simulink model "NominalEncounter"  (R2018b)
settings: Solver=ode45  StartTime=0.0  StopTime=600  RelTol=1e-3  EnableMultiTasking=on
libraries: simulink x4, CalcMinDist x3, NominalTrajectory x2, BasicAircraftDynamicsBlock x2, FlattenAircraftEstimateBus x2, PerfectSurveillanceBlock x2, SLoWCBlock x1, WellClearMetricsBlock x1, StopConditionsBlock x1
settings Model: Creator=JO20596  LastModifiedBy=BI28030
settings DataIOCC: LimitDataPoints=on  MaxDataPoints=10000  SignalLoggingSaveFormat=ModelDataLogs  SaveState=on  StateSaveName=xoutNew  OutputSaveName=youtNew
settings OptimizationCC: ExpressionDepthLimit=2147483647  LifeSpan=inf
settings DebuggingCC: UnderspecifiedInitializationDetection=Classic  MergeDetectMultiDrivingBlocksExec=none  SolverPrmCheckMsg=warning  FcnCallInpInsideContextMsg=warning  StateNameClashWarn=warning  SFUnexpectedBacktrackingDiag=warning  SFNoUnconditionalDefaultTransitionDiag=warning  SFExecutionAtInitializationDiag=none
settings HardwareCC: ProdBitPerPointer=32  ProdBitPerSizeT=32  ProdBitPerPtrDiffT=32  ProdLargestAtomicFloat=None  ProdIntDivRoundTo=Undefined  ProdEndianess=Unspecified  ProdWordSize=32  ProdHWDeviceType=32-bit Generic
settings ModelReferenceCC: PropagateSignalLabelsOutOfModel=off
settings SFSimCC: SimUseLocalCustomCode=off
settings RTWCC: RTWUseLocalCustomCode=off
settings CodeAppCC: StateflowObjectComments=on
settings GRTTargetCC: TargetLangStandard=C89/C90 (ANSI)  GeneratePreprocessorConditionals=Disable all  CombineOutputUpdateFcns=off  GRTInterface=on
settings ConfigComp: CovMetricSettings=dw  CovHtmlReporting=on  CovSaveCumulativeToWorkspaceVar=on  CovSaveSingleToWorkspaceVar=on  CovExternalEMLEnable=off

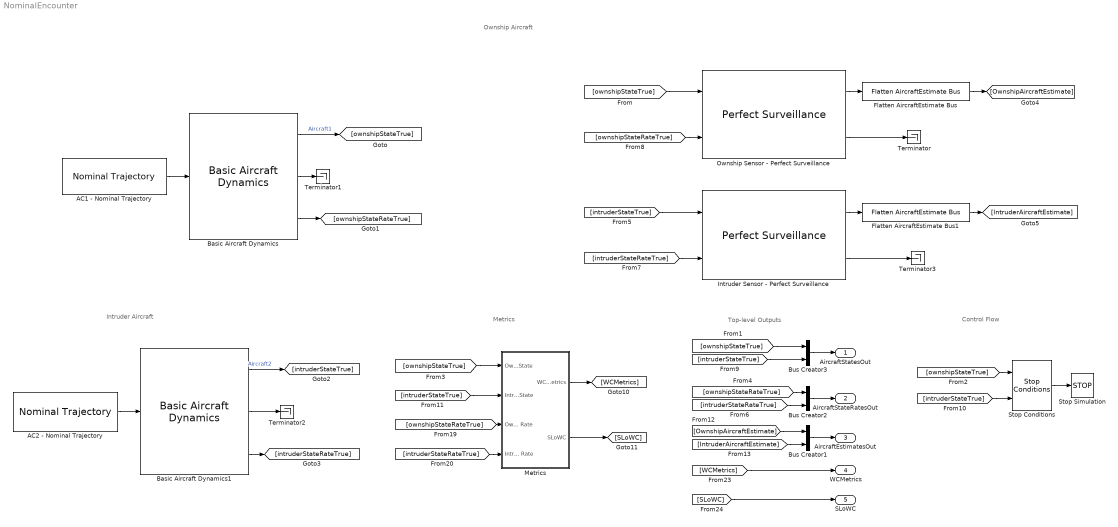
== system NominalEncounter ==
  note: Metrics
  note: Control Flow
  note: Top-level Outputs
  note: Ownship Aircraft
  note: Intruder Aircraft
  AC1 - Nominal Trajectory : NominalTrajectory/Nominal Trajectory  eventFilename=event1.mat  ts=.1
  AC2 - Nominal Trajectory : NominalTrajectory/Nominal Trajectory  eventFilename=event2.mat  ts=.1
  Basic Aircraft Dynamics : BasicAircraftDynamicsBlock/Basic Aircraft Dynamics  ts_dynamics=.1  v_ftps_0=ac1dyn_v_ftps  N_ft_0=ac1dyn_N_ft  E_ft_0=ac1dyn_E_ft  h_ft_0=ac1dyn_h_ft  psi_rad_0=ac1dyn_psi_rad  theta_rad_0=ac1dyn_theta_rad  phi_rad_0=ac1dyn_phi_rad  a_ftpss_0=ac1dyn_a_ftpss  v_ftps_max=ac1dyn_con.maxAirspeed_ftps  v_ftps_min=ac1dyn_con.minAirspeed_ftps  dv_ftpss_max=ac1dyn_con.maxAcceleration_ftpss  dv_ftpss_min=ac1dyn_con.minAcceleration_ftpss  dh_ftps_max=ac1dyn_con.maxVerticalRate_ftps  dh_ftps_min=ac1dyn_con.minVerticalRate_ftps  q_radps_max=ac1dyn_con.maxPitchRate_radps  phi_rad_max=ac1dyn_con.maxBankAngle_rad  dphi_radps_max=ac1dyn_con.maxRollRate_radps  r_radps_max=ac1dyn_con.maxYawRate_radps  pNUM=ac1dyn_con.dynamicsNumeratorRollRate  pDEN=ac1dyn_con.dynamicsDenominatorRollRate  hNUM=ac1dyn_con.dynamicsNumeratorVerticalRate  hDEN=ac1dyn_con.dynamicsDenominatorVerticalRate  rNUM=ac1dyn_con.dynamicsNumeratorYawRate  rDEN=ac1dyn_con.dynamicsDenominatorYawRate  lat0_rad=ac1dyn_lat0_rad  lon0_rad=ac1dyn_lon0_rad  alt_ft=ac1dyn_alt0_ft
  Basic Aircraft Dynamics1 : BasicAircraftDynamicsBlock/Basic Aircraft Dynamics  ts_dynamics=.1  v_ftps_0=ac2dyn_v_ftps  N_ft_0=ac2dyn_N_ft  E_ft_0=ac2dyn_E_ft  h_ft_0=ac2dyn_h_ft  psi_rad_0=ac2dyn_psi_rad  theta_rad_0=ac2dyn_theta_rad  phi_rad_0=ac2dyn_phi_rad  a_ftpss_0=ac2dyn_a_ftpss  v_ftps_max=ac2dyn_con.maxAirspeed_ftps  v_ftps_min=ac2dyn_con.minAirspeed_ftps  dv_ftpss_max=ac2dyn_con.maxAcceleration_ftpss  dv_ftpss_min=ac2dyn_con.minAcceleration_ftpss  dh_ftps_max=ac2dyn_con.maxVerticalRate_ftps  dh_ftps_min=ac2dyn_con.minVerticalRate_ftps  q_radps_max=ac2dyn_con.maxPitchRate_radps  phi_rad_max=ac2dyn_con.maxBankAngle_rad  dphi_radps_max=ac2dyn_con.maxRollRate_radps  r_radps_max=ac2dyn_con.maxYawRate_radps  pNUM=ac2dyn_con.dynamicsNumeratorRollRate  pDEN=ac2dyn_con.dynamicsDenominatorRollRate  hNUM=ac2dyn_con.dynamicsNumeratorVerticalRate  hDEN=ac2dyn_con.dynamicsDenominatorVerticalRate  rNUM=ac2dyn_con.dynamicsNumeratorYawRate  rDEN=ac2dyn_con.dynamicsDenominatorYawRate  lat0_rad=ac2dyn_lat0_rad  lon0_rad=ac2dyn_lon0_rad  alt_ft=ac2dyn_alt0_ft
  Bus Creator1 : BusCreator  Inputs=2
  Bus Creator2 : BusCreator  Inputs=2
  Bus Creator3 : BusCreator  Inputs=2
  Flatten AircraftEstimate Bus : FlattenAircraftEstimateBus/Flatten AircraftEstimate Bus  SystemSampleTime=-1
  Flatten AircraftEstimate Bus1 : FlattenAircraftEstimateBus/Flatten AircraftEstimate Bus  SystemSampleTime=-1
  Intruder Sensor - Perfect Surveillance : PerfectSurveillanceBlock/Perfect Surveillance  Description=|  dt=ac1IntPerfSurv_surveillanceSampletime_s
      | Documentation for Perfect Observation Block                                                                                                                                                                                                                                                                                                                                                                                                          
      |                                                                                                                                                                                                                                                                                                                                                                                                                                                      
      | Description:  The perfect observation block, also known as a perfect                                                                                                                                                                                                                                                                                                                                                                                 
      | surveillance block, receives an Aircraft State, nominally from a Basic                                                                                                                                                                                                                                                                                                                                                                               
      | Aircraft Dynamics block, and outputs an Aircraft Estimate.  The Aircraft                                                                                                                                                                                                                                                                                                                                                                             
      | State that is received as input consists of Latitude, Longitude, and                                                                                                                                                                                                                                                                                                                                                                                 
      | Altitude state information as well as the aircraft position in local                                                                                                                                                                                                                                                                                                                                                                                 
      | coordinates in units of feet for north, east, and height.  The Aircraft                                                                                                                                                                                                                                                                                                                                                                              
      | Estimate outputs consist of estimates for the aircraft Latitude, Longitude, and Altitude, the east, north up position, and sensor covariance.  For perfect surveillance, the covariance estimates are all set to zero as default.  In addition, "time of validity" and a Boolean flag for the sensor report, "is Valid", are outputted as part of the Aircraft Estimate.                                                                             
      |                                                                                                                                                                                                                                                                                                                                                                                                                                                      
      | The initial perfect surveillance block developed receives the aircraft state information from the "AC2 - Basic Aircraft Dynamics" block within the "nominalEncounter" study.  Since the expected output from the AC1 and AC2 aircraft states have slightly different output parameters than what is provided from the perfect surveillance block (i.e., covariance estimates, isValid, and time of validity), the perfect surveillance block         
      | AircraftEstimate output has been left disconnected.                                                                                                                                                                                                                                                                                                                                                                                                  
      |                                                                                                                                                                                                                                                                                                                                                                                                                                                      
      | The initial unit test performed for this perfect observation block was to                                                                                                                                                                                                                                                                                                                                                                            
      | run the nominalEncounter study and to ensure that the simulation completes and no exceptions are encountered.  This unit test was successful (other than receiving a warning that the output of the perfect surveillance block is not connected, which was expected).  A more comprehensive future unit test would be to evaluate the position inputs and compare them with the position outputs to ensure that they are consistent with one another.
  Metrics : Subsystem
  Ownship Sensor - Perfect Surveillance : PerfectSurveillanceBlock/Perfect Surveillance  Description=|  dt=ac1OwnPerfSurv_surveillanceSampletime_s
      | Documentation for Perfect Observation Block                                                                                                                                                                                                                                                                                                                                                                                                          
      |                                                                                                                                                                                                                                                                                                                                                                                                                                                      
      | Description:  The perfect observation block, also known as a perfect                                                                                                                                                                                                                                                                                                                                                                                 
      | surveillance block, receives an Aircraft State, nominally from a Basic                                                                                                                                                                                                                                                                                                                                                                               
      | Aircraft Dynamics block, and outputs an Aircraft Estimate.  The Aircraft                                                                                                                                                                                                                                                                                                                                                                             
      | State that is received as input consists of Latitude, Longitude, and                                                                                                                                                                                                                                                                                                                                                                                 
      | Altitude state information as well as the aircraft position in local                                                                                                                                                                                                                                                                                                                                                                                 
      | coordinates in units of feet for north, east, and height.  The Aircraft                                                                                                                                                                                                                                                                                                                                                                              
      | Estimate outputs consist of estimates for the aircraft Latitude, Longitude, and Altitude, the east, north up position, and sensor covariance.  For perfect surveillance, the covariance estimates are all set to zero as default.  In addition, "time of validity" and a Boolean flag for the sensor report, "is Valid", are outputted as part of the Aircraft Estimate.                                                                             
      |                                                                                                                                                                                                                                                                                                                                                                                                                                                      
      | The initial perfect surveillance block developed receives the aircraft state information from the "AC2 - Basic Aircraft Dynamics" block within the "nominalEncounter" study.  Since the expected output from the AC1 and AC2 aircraft states have slightly different output parameters than what is provided from the perfect surveillance block (i.e., covariance estimates, isValid, and time of validity), the perfect surveillance block         
      | AircraftEstimate output has been left disconnected.                                                                                                                                                                                                                                                                                                                                                                                                  
      |                                                                                                                                                                                                                                                                                                                                                                                                                                                      
      | The initial unit test performed for this perfect observation block was to                                                                                                                                                                                                                                                                                                                                                                            
      | run the nominalEncounter study and to ensure that the simulation completes and no exceptions are encountered.  This unit test was successful (other than receiving a warning that the output of the perfect surveillance block is not connected, which was expected).  A more comprehensive future unit test would be to evaluate the position inputs and compare them with the position outputs to ensure that they are consistent with one another.
  Stop Conditions : StopConditionsBlock/Stop Conditions  range_limit_ft=stop_range_ft  altitude_limit_ft=stop_altitude_ft
  Stop Simulation : Stop
  Terminator{,1..3} (4 alike) : Terminator
  AircraftStatesOut : Outport
  AircraftStateRatesOut : Outport  Port=2
  AircraftEstimatesOut : Outport  Port=3
  WCMetrics : Outport  Port=4
  SLoWC : Outport  Port=5
  wires:
  Bus Creator2/1 -> AircraftStateRatesOut/1
  Stop Conditions/1 -> Stop Simulation/1
  [ownshipStateTrue] -> Stop Conditions/1
  [ownshipStateRateTrue] -> Bus Creator2/1
  [intruderStateRateTrue] -> Bus Creator2/2
  [intruderStateTrue] -> Stop Conditions/2
  [ownshipStateTrue] -> Metrics/1(Ownship State)
  [intruderStateTrue] -> Metrics/2(Intruder State)
  [ownshipStateRateTrue] -> Metrics/3(Ownship State Rate)
  [intruderStateRateTrue] -> Metrics/4(Intruder State Rate)
  Metrics/1(WCMetrics) -> [WCMetrics]
  Metrics/2(SLoWC) -> [SLoWC]
  [WCMetrics] -> WCMetrics/1
  [SLoWC] -> SLoWC/1
  Basic Aircraft Dynamics1/3 -> [intruderStateRateTrue]
  Basic Aircraft Dynamics/2 -> Terminator1/1
  AC1 - Nominal Trajectory/1 -> Basic Aircraft Dynamics/1
  Basic Aircraft Dynamics1/1 -> [intruderStateTrue]  "Aircraft2"
  Basic Aircraft Dynamics1/2 -> Terminator2/1
  AC2 - Nominal Trajectory/1 -> Basic Aircraft Dynamics1/1
  Basic Aircraft Dynamics/1 -> [ownshipStateTrue]  "Aircraft1"
  [ownshipStateTrue] -> Ownship Sensor - Perfect Surveillance/1
  Basic Aircraft Dynamics/3 -> [ownshipStateRateTrue]
  [intruderStateTrue] -> Intruder Sensor - Perfect Surveillance/1
  [intruderStateRateTrue] -> Intruder Sensor - Perfect Surveillance/2
  [ownshipStateRateTrue] -> Ownship Sensor - Perfect Surveillance/2
  [OwnshipAircraftEstimate] -> Bus Creator1/1
  [IntruderAircraftEstimate] -> Bus Creator1/2
  Ownship Sensor - Perfect Surveillance/1 -> Flatten AircraftEstimate Bus/1
  Intruder Sensor - Perfect Surveillance/1 -> Flatten AircraftEstimate Bus1/1
  Bus Creator1/1 -> AircraftEstimatesOut/1
  Flatten AircraftEstimate Bus1/1 -> [IntruderAircraftEstimate]
  Flatten AircraftEstimate Bus/1 -> [OwnshipAircraftEstimate]
  [ownshipStateTrue] -> Bus Creator3/1
  [intruderStateTrue] -> Bus Creator3/2
  Bus Creator3/1 -> AircraftStatesOut/1
  Ownship Sensor - Perfect Surveillance/2 -> Terminator/1
  Intruder Sensor - Perfect Surveillance/2 -> Terminator3/1

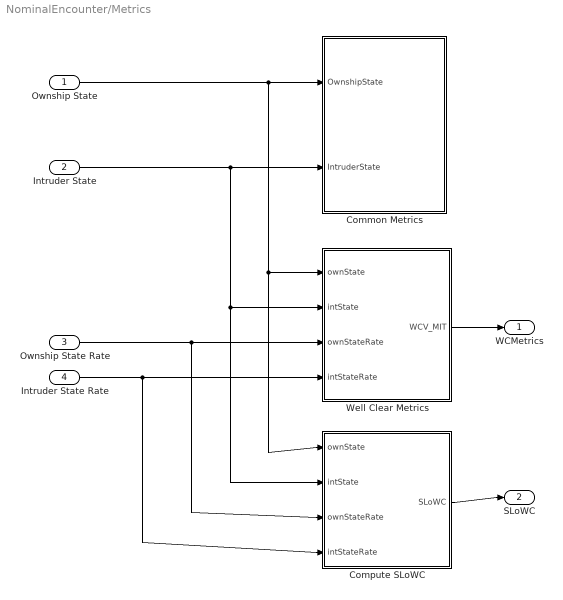
== system NominalEncounter/Metrics ==
  Ownship State : Inport
  Intruder State : Inport  Port=2
  Ownship State Rate : Inport  Port=3
  Intruder State Rate : Inport  Port=4
  Common Metrics : Subsystem  AncestorBlock=CommonMetricsBlock/Common Metrics  mask(CommonMetrics){}
      mask help:
      | Calculates metrics common to all aircraft encounters, those having to do with the separation
      | between aircraft. Metrics pertaining to the operation of advisory systems (e.g. alert rate) are not
      | included in this block.
      |
      | The calculated metrics are saved to a workspace.
      mask Help:
      | Calculates metrics common to all aircraft encounters, those having to do with the separation
      | between aircraft. Metrics pertaining to the operation of advisory systems (e.g. alert rate) are not
      | included in this block.
      | 
      | The calculated metrics are saved to a workspace.
      | 
      | INPUTS
      | ==========
      | Aircraft1 - A CASSATT v6 AircraftState bus from first aircraft
      | Aircraft2 - A CASSATT v6 AircraftState bus from second aircraft
      | 
      | OUTPUTS (Saved to Workspace)
      | ==========
      | NMAC - Near Mid Air Collision.  True if the separation between the two
      |     aircraft has ever been simultaneously less than 100 feet vertically and
      |     500 feet horizontally.
      | hmd_ft - Horizontal Miss Distance in feet.  The minimum horizontal
      |     separation that has occurred between the two aircraft.
      | vmd_ft - Vertical Miss Distance in feet.  The vertical separation of the
      |     two aircaft at the Time of Closest Approach.
      | tca - Time of Closest Approach in seconds.  Prior to horizontal separation
      |     of less than 500 feet, the Time of Closest Approach is the time when
      |     the minimum horizontal separation was achieved.  Once horizontal
      |     separation has been less than 500 feet, the Time of Closest Approach is
      |     when minimum vertical separation occurs while horizontal separation is
      |     less than 500 feet.
  Compute SLoWC : Subsystem  mask{DMOD=4000, tauMod=35, altDiff=450}
      mask prompts: altDiff "Altitude Difference Threshold:"
  Well Clear Metrics : Subsystem
  WCMetrics : Outport
  SLoWC : Outport  Port=2
  wires:
  Ownship State/1 -> Common Metrics/1(OwnshipState), Well Clear Metrics/1(ownState), Compute SLoWC/1(ownState)
  Intruder State/1 -> Common Metrics/2(IntruderState), Well Clear Metrics/2(intState), Compute SLoWC/2(intState)
  Ownship State Rate/1 -> Well Clear Metrics/3(ownStateRate), Compute SLoWC/3(ownStateRate)
  Intruder State Rate/1 -> Well Clear Metrics/4(intStateRate), Compute SLoWC/4(intStateRate)
  Well Clear Metrics/1(WCV_MIT) -> WCMetrics/1
  Compute SLoWC/1(SLoWC) -> SLoWC/1

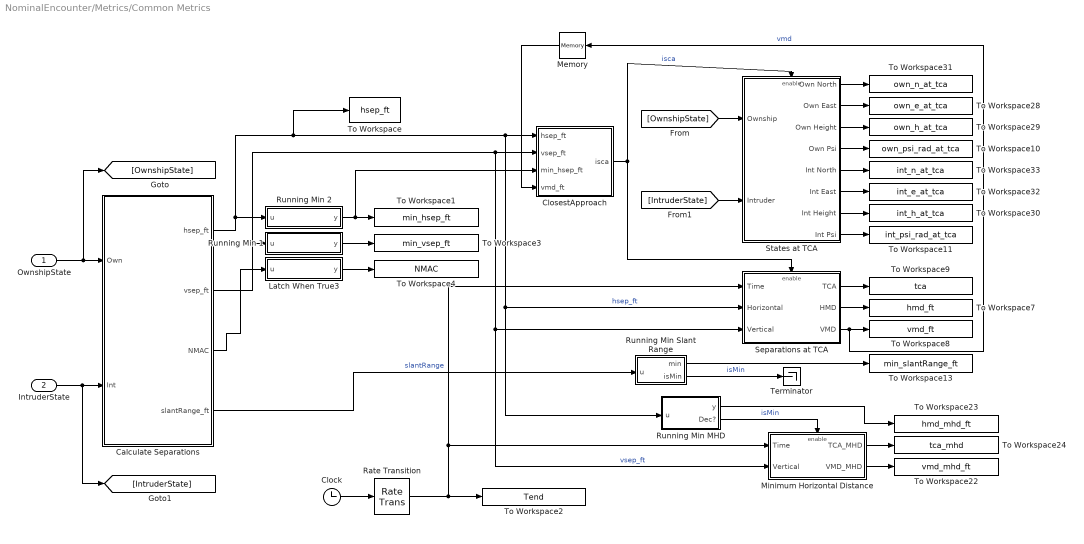
== system NominalEncounter/Metrics/Common Metrics ==
  OwnshipState : Inport  OutDataTypeStr=Bus: AircraftState  PortDimensions=1
  IntruderState : Inport  Port=2  OutDataTypeStr=Bus: AircraftState  PortDimensions=1
  Calculate Separations : Subsystem
  Clock : Clock
  ClosestApproach : Subsystem
  Latch When True3 : Subsystem
      mask Display: disp('Latch when true')
  Memory : Memory
  Minimum Horizontal Distance : Subsystem  TreatAsAtomicUnit=on
  Rate Transition : RateTransition
  Running Min 1 : Subsystem
      mask Display: disp('Running min')
  Running Min 2 : Subsystem
      mask Display: disp('Running min')
  Running Min MHD : Subsystem
  Running Min Slant Range : Subsystem
  Separations at TCA : Subsystem  TreatAsAtomicUnit=on
  States at TCA : Subsystem  TreatAsAtomicUnit=on
  Terminator : Terminator
  To Workspace : ToWorkspace  VariableName=hsep_ft  SaveFormat=Timeseries  SampleTime=-1
  To Workspace1 : ToWorkspace  VariableName=min_hsep_ft  SampleTime=-1
      settings: MaxDataPoints=1
  To Workspace10 : ToWorkspace  VariableName=own_psi_rad_at_tca  SampleTime=-1
      settings: MaxDataPoints=1
  To Workspace11 : ToWorkspace  VariableName=int_psi_rad_at_tca  SampleTime=-1
      settings: MaxDataPoints=1
  To Workspace13 : ToWorkspace  VariableName=min_slantRange_ft  SampleTime=-1
      settings: MaxDataPoints=1
  To Workspace2 : ToWorkspace  VariableName=Tend  SampleTime=-1
      settings: MaxDataPoints=1
  To Workspace22 : ToWorkspace  VariableName=vmd_mhd_ft  SampleTime=-1
      settings: MaxDataPoints=1
  To Workspace23 : ToWorkspace  VariableName=hmd_mhd_ft  SampleTime=-1
      settings: MaxDataPoints=1
  To Workspace24 : ToWorkspace  VariableName=tca_mhd  SampleTime=-1
      settings: MaxDataPoints=1
  To Workspace28 : ToWorkspace  VariableName=own_e_at_tca  SampleTime=-1
      settings: MaxDataPoints=1
  To Workspace29 : ToWorkspace  VariableName=own_h_at_tca  SampleTime=-1
      settings: MaxDataPoints=1
  To Workspace3 : ToWorkspace  VariableName=min_vsep_ft  SampleTime=-1
      settings: MaxDataPoints=1
  To Workspace30 : ToWorkspace  VariableName=int_h_at_tca  SampleTime=-1
      settings: MaxDataPoints=1
  To Workspace31 : ToWorkspace  VariableName=own_n_at_tca  SampleTime=-1
      settings: MaxDataPoints=1
  To Workspace32 : ToWorkspace  VariableName=int_e_at_tca  SampleTime=-1
      settings: MaxDataPoints=1
  To Workspace33 : ToWorkspace  VariableName=int_n_at_tca  SampleTime=-1
      settings: MaxDataPoints=1
  To Workspace4 : ToWorkspace  VariableName=NMAC  SampleTime=-1
      settings: MaxDataPoints=1
  To Workspace7 : ToWorkspace  VariableName=hmd_ft  SampleTime=-1
      settings: MaxDataPoints=1
  To Workspace8 : ToWorkspace  VariableName=vmd_ft  SampleTime=-1
      settings: MaxDataPoints=1
  To Workspace9 : ToWorkspace  VariableName=tca  SampleTime=-1
      settings: MaxDataPoints=1
  wires:
  Calculate Separations/2(vsep_ft) -> ClosestApproach/2(vsep_ft), Separations at TCA/3(Vertical), Minimum Horizontal Distance/2(Vertical), Running Min 1/1(u)  "vsep_ft"
  Rate Transition/1 -> To Workspace2/1, Separations at TCA/1(Time), Minimum Horizontal Distance/1(Time)
  Minimum Horizontal Distance/1(TCA_MHD) -> To Workspace24/1
  Minimum Horizontal Distance/2(VMD_MHD) -> To Workspace22/1
  Running Min MHD/1(y) -> To Workspace23/1
  Running Min MHD/2(Dec?) -> Minimum Horizontal Distance/Enable  "isMin"
  Running Min Slant Range/2(isMin) -> Terminator/1  "isMin"
  Running Min 2/1(y) -> To Workspace1/1, ClosestApproach/3(min_hsep_ft)
  Separations at TCA/3(VMD) -> To Workspace8/1, Memory/1  "vmd"
  Clock/1 -> Rate Transition/1
  Separations at TCA/1(TCA) -> To Workspace9/1
  Latch When True3/1(y) -> To Workspace4/1
  IntruderState/1 -> Calculate Separations/2(Int), [IntruderState]
  Calculate Separations/3(NMAC) -> Latch When True3/1(u)
  Separations at TCA/2(HMD) -> To Workspace7/1
  Running Min 1/1(y) -> To Workspace3/1
  Calculate Separations/4(slantRange_ft) -> Running Min Slant Range/1(u)  "slantRange"
  Running Min Slant Range/1(min) -> To Workspace13/1
  Calculate Separations/1(hsep_ft) -> Running Min 2/1(u), To Workspace/1, ClosestApproach/1(hsep_ft), Separations at TCA/2(Horizontal), Running Min MHD/1(u)  "hsep_ft"
  ClosestApproach/1(isca) -> Separations at TCA/Enable, States at TCA/Enable  "isca"
  States at TCA/1(Own North) -> To Workspace31/1
  States at TCA/2(Own East) -> To Workspace28/1
  States at TCA/3(Own Height) -> To Workspace29/1
  States at TCA/5(Int North) -> To Workspace33/1
  States at TCA/6(Int East) -> To Workspace32/1
  States at TCA/7(Int Height) -> To Workspace30/1
  [OwnshipState] -> States at TCA/1(Ownship)
  [IntruderState] -> States at TCA/2(Intruder)
  OwnshipState/1 -> Calculate Separations/1(Own), [OwnshipState]
  Memory/1 -> ClosestApproach/4(vmd_ft)
  States at TCA/4(Own Psi) -> To Workspace10/1
  States at TCA/8(Int Psi) -> To Workspace11/1

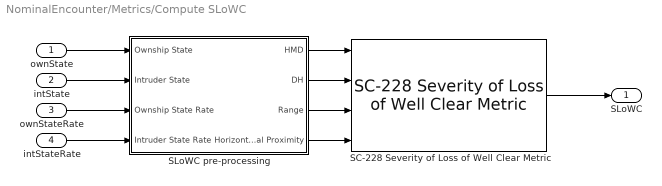
== system NominalEncounter/Metrics/Compute SLoWC ==
  ownState : Inport
  intState : Inport  Port=2
  ownStateRate : Inport  Port=3
  intStateRate : Inport  Port=4
  SC-228 Severity of Loss of Well Clear Metric : SLoWCBlock/SC-228 Severity of Loss of Well Clear Metric  DMOD=DMOD  altDiffThreshold=altDiff
  SLoWC pre-processing : Subsystem
  SLoWC : Outport
  wires:
  SLoWC pre-processing/2(DH) -> SC-228 Severity of Loss of Well Clear Metric/2
  SC-228 Severity of Loss of Well Clear Metric/1 -> SLoWC/1
  SLoWC pre-processing/1(HMD) -> SC-228 Severity of Loss of Well Clear Metric/1
  ownState/1 -> SLoWC pre-processing/1(Ownship State)
  SLoWC pre-processing/4(Horizontal Proximity) -> SC-228 Severity of Loss of Well Clear Metric/4
  SLoWC pre-processing/3(Range) -> SC-228 Severity of Loss of Well Clear Metric/3
  intState/1 -> SLoWC pre-processing/2(Intruder State)
  intStateRate/1 -> SLoWC pre-processing/4(Intruder State Rate)
  ownStateRate/1 -> SLoWC pre-processing/3(Ownship State Rate)

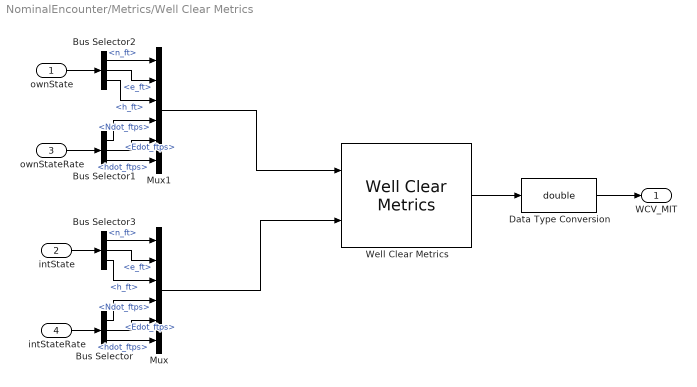
== system NominalEncounter/Metrics/Well Clear Metrics ==
  ownState : Inport  OutDataTypeStr=Bus: AircraftState
  intState : Inport  Port=2  OutDataTypeStr=Bus: AircraftState
  ownStateRate : Inport  Port=3  OutDataTypeStr=Bus: AircraftStateRate
  intStateRate : Inport  Port=4  OutDataTypeStr=Bus: AircraftStateRate
  Bus Selector : BusSelector  OutputSignals=Ndot_ftps,Edot_ftps,hdot_ftps
  Bus Selector1 : BusSelector  OutputSignals=Ndot_ftps,Edot_ftps,hdot_ftps
  Bus Selector2 : BusSelector  OutputSignals=n_ft,e_ft,h_ft
  Bus Selector3 : BusSelector  OutputSignals=n_ft,e_ft,h_ft
  Data Type Conversion : DataTypeConversion  OutDataTypeStr=double
  Mux : Mux  Inputs=6
  Mux1 : Mux  Inputs=6
  Well Clear Metrics : WellClearMetricsBlock/Well Clear Metrics  tauThreshold=wcm_modTau  hmdThreshold=wcm_HMD  tauVThreshold=wcm_TOCA  altThreshold=wcm_altThresh  rngThreshold=wcm_rangeThresh
  WCV_MIT : Outport
  wires:
  Well Clear Metrics/1 -> Data Type Conversion/1
  intStateRate/1 -> Bus Selector/1
  ownStateRate/1 -> Bus Selector1/1
  ownState/1 -> Bus Selector2/1
  intState/1 -> Bus Selector3/1
  Bus Selector3/1 -> Mux/1  "<n_ft>"
  Bus Selector3/2 -> Mux/2  "<e_ft>"
  Bus Selector3/3 -> Mux/3  "<h_ft>"
  Bus Selector/1 -> Mux/4  "<Ndot_ftps>"
  Bus Selector/2 -> Mux/5  "<Edot_ftps>"
  Bus Selector/3 -> Mux/6  "<hdot_ftps>"
  Bus Selector2/1 -> Mux1/1  "<n_ft>"
  Bus Selector2/2 -> Mux1/2  "<e_ft>"
  Bus Selector2/3 -> Mux1/3  "<h_ft>"
  Bus Selector1/3 -> Mux1/6  "<hdot_ftps>"
  Bus Selector1/1 -> Mux1/4  "<Ndot_ftps>"
  Bus Selector1/2 -> Mux1/5  "<Edot_ftps>"
  Mux1/1 -> Well Clear Metrics/1
  Mux/1 -> Well Clear Metrics/2
  Data Type Conversion/1 -> WCV_MIT/1

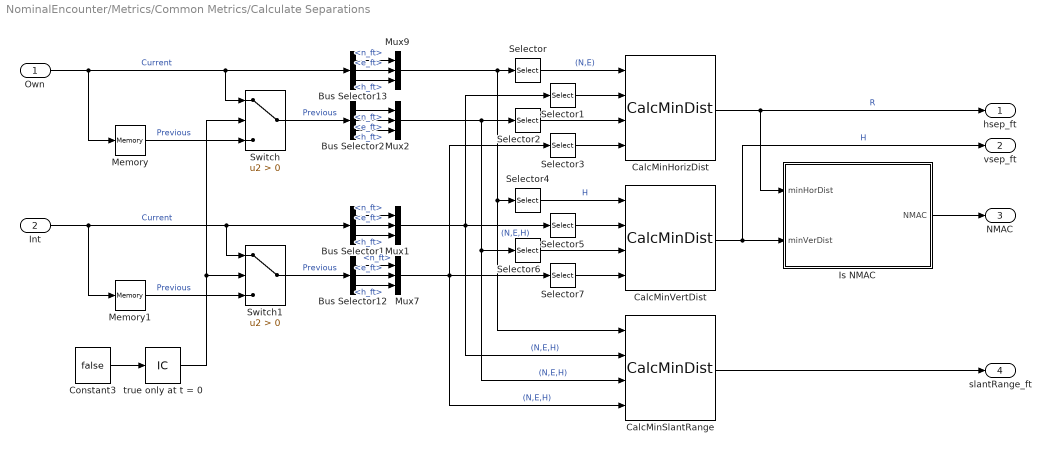
== system NominalEncounter/Metrics/Common Metrics/Calculate Separations ==
  Own : Inport
  Int : Inport  Port=2
  Bus Selector{1..2,12..13} (4 alike) : BusSelector  OutputSignals=n_ft,e_ft,h_ft
  CalcMinHorizDist : CalcMinDist/CalcMinDist
      settings: SourceProductName=CASSATTv6: Metrics Library
  CalcMinSlantRange : CalcMinDist/CalcMinDist
      settings: SourceProductName=CASSATTv6: Metrics Library
  CalcMinVertDist : CalcMinDist/CalcMinDist
      settings: SourceProductName=CASSATTv6: Metrics Library
  Constant3 : Constant  Value=false  SampleTime=Inf
  Is NMAC : Subsystem
  Memory : Memory
  Memory1 : Memory
  Mux{1..2,7,9} (4 alike) : Mux  Inputs=3
  Selector{,1..3} (4 alike) : Selector  InputPortWidth=3  IndexOptions=Index vector (dialog)  Indices=[1 2]  OutputSizes=1
  Selector{4..7} (4 alike) : Selector  InputPortWidth=3  IndexOptions=Index vector (dialog)  Indices=3  OutputSizes=1
  Switch : Switch  Criteria=u2 > Threshold
  Switch1 : Switch  Criteria=u2 > Threshold
  true only at t = 0 : InitialCondition  Value=true
  hsep_ft : Outport
  vsep_ft : Outport  Port=2
  NMAC : Outport  Port=3
  slantRange_ft : Outport  Port=4
  wires:
  CalcMinHorizDist/1 -> Is NMAC/1(minHorDist), hsep_ft/1  "R"
  true only at t = 0/1 -> Switch/2, Switch1/2
  Constant3/1 -> true only at t = 0/1
  Memory1/1 -> Switch1/3  "Previous"
  Memory/1 -> Switch/3  "Previous"
  Mux9/1 -> Selector/1, Selector4/1, CalcMinSlantRange/1  "(N,E,H)"
  Bus Selector12/2 -> Mux7/2  "<e_ft>"
  Bus Selector12/1 -> Mux7/1  "<n_ft>"
  Bus Selector12/3 -> Mux7/3  "<h_ft>"
  Mux7/1 -> Selector3/1, Selector7/1, CalcMinSlantRange/4  "(N,E,H)"
  CalcMinSlantRange/1 -> slantRange_ft/1
  Int/1 -> Bus Selector1/1, Switch1/1, Memory1/1  "Current"
  Own/1 -> Memory/1, Bus Selector13/1, Switch/1  "Current"
  Switch1/1 -> Bus Selector12/1  "Previous"
  CalcMinVertDist/1 -> vsep_ft/1, Is NMAC/2(minVerDist)  "H"
  Bus Selector13/1 -> Mux9/1  "<n_ft>"
  Bus Selector13/2 -> Mux9/2  "<e_ft>"
  Bus Selector13/3 -> Mux9/3  "<h_ft>"
  Bus Selector1/1 -> Mux1/1  "<n_ft>"
  Bus Selector1/2 -> Mux1/2  "<e_ft>"
  Bus Selector1/3 -> Mux1/3  "<h_ft>"
  Switch/1 -> Bus Selector2/1  "Previous"
  Bus Selector2/1 -> Mux2/1  "<n_ft>"
  Bus Selector2/2 -> Mux2/2  "<e_ft>"
  Bus Selector2/3 -> Mux2/3  "<h_ft>"
  Mux1/1 -> Selector1/1, Selector5/1, CalcMinSlantRange/2  "(N,E,H)"
  Mux2/1 -> Selector6/1, CalcMinSlantRange/3, Selector2/1  "(N,E,H)"
  Selector/1 -> CalcMinHorizDist/1  "(N,E)"
  Selector1/1 -> CalcMinHorizDist/2
  Selector2/1 -> CalcMinHorizDist/3
  Selector3/1 -> CalcMinHorizDist/4
  Selector4/1 -> CalcMinVertDist/1  "H"
  Selector5/1 -> CalcMinVertDist/2
  Selector6/1 -> CalcMinVertDist/3
  Selector7/1 -> CalcMinVertDist/4
  Is NMAC/1(NMAC) -> NMAC/1

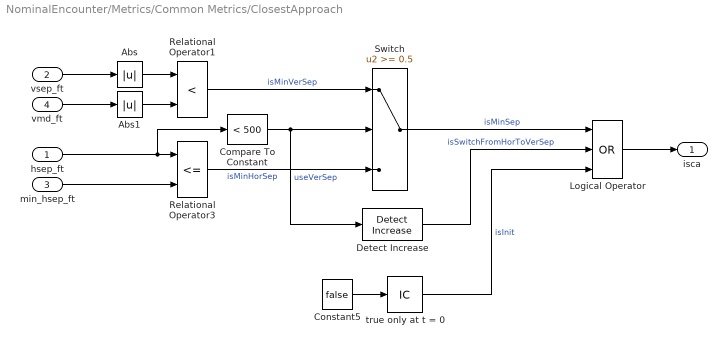
== system NominalEncounter/Metrics/Common Metrics/ClosestApproach ==
  hsep_ft : Inport
  vsep_ft : Inport  Port=2
  min_hsep_ft : Inport  Port=3
  vmd_ft : Inport  Port=4
  Abs : Abs
  Abs1 : Abs
  Compare To Constant : simulink/Logic and Bit Operations/Compare To Constant  relop=<  const=500  OutDataTypeStr=boolean
  Constant5 : Constant  Value=false  SampleTime=Inf
  Detect Increase : simulink/Logic and Bit Operations/Detect Increase  vinit=0.0  OutDataTypeStr=boolean
  Logical Operator : Logic  Operator=OR  Inputs=3  AllPortsSameDT=off  OutDataTypeStr=boolean
  Relational Operator1 : RelationalOperator  Operator=<  OutDataTypeStr=boolean  RndMeth=Nearest
  Relational Operator3 : RelationalOperator  Operator=<=  OutDataTypeStr=boolean  RndMeth=Nearest
  Switch : Switch  Threshold=0.5
  true only at t = 0 : InitialCondition  Value=true
  isca : Outport
  wires:
  Detect Increase/1 -> Logical Operator/2  "isSwitchFromHorToVerSep"
  Logical Operator/1 -> isca/1
  hsep_ft/1 -> Compare To Constant/1, Relational Operator3/1
  Compare To Constant/1 -> Switch/2, Detect Increase/1  "useVerSep"
  Switch/1 -> Logical Operator/1  "isMinSep"
  vsep_ft/1 -> Abs/1
  vmd_ft/1 -> Abs1/1
  Abs1/1 -> Relational Operator1/2
  Abs/1 -> Relational Operator1/1
  Relational Operator1/1 -> Switch/1  "isMinVerSep"
  min_hsep_ft/1 -> Relational Operator3/2
  Relational Operator3/1 -> Switch/3  "isMinHorSep"
  Constant5/1 -> true only at t = 0/1
  true only at t = 0/1 -> Logical Operator/3  "isInit"

== system NominalEncounter/Metrics/Common Metrics/Latch When True3 ==
  u : Inport  PortDimensions=1
  Logical Operator : Logic  Operator=OR  AllPortsSameDT=off  OutDataTypeStr=boolean
  Unit Delay : UnitDelay  SampleTime=-1
  y : Outport
  wires:
  Unit Delay/1 -> Logical Operator/2
  Logical Operator/1 -> Unit Delay/1, y/1
  u/1 -> Logical Operator/1

== system NominalEncounter/Metrics/Common Metrics/Minimum Horizontal Distance ==
  note: This subsytems passes the input signal through whenever the enable signal is true. The output is held when the enable signal is false.
  Time : Inport
  Vertical : Inport  Port=2
  isca : EnablePort
  TCA_MHD : Outport
  VMD_MHD : Outport  Port=2
  wires:
  Vertical/1 -> VMD_MHD/1
  Time/1 -> TCA_MHD/1

== system NominalEncounter/Metrics/Common Metrics/Running Min 1 ==
  u : Inport  PortDimensions=1
  MinMax : MinMax  Inputs=2
  Unit Delay : UnitDelay  InitialCondition=NaN  SampleTime=-1
  y : Outport
  wires:
  u/1 -> MinMax/1
  MinMax/1 -> y/1, Unit Delay/1
  Unit Delay/1 -> MinMax/2

== system NominalEncounter/Metrics/Common Metrics/Running Min 2 ==
  u : Inport  PortDimensions=1
  MinMax : MinMax  Inputs=2
  Unit Delay : UnitDelay  InitialCondition=NaN  SampleTime=-1
  y : Outport
  wires:
  Unit Delay/1 -> MinMax/2
  MinMax/1 -> Unit Delay/1, y/1
  u/1 -> MinMax/1

== system NominalEncounter/Metrics/Common Metrics/Running Min MHD ==
  u : Inport
  Memory : Memory  InitialCondition=42000000
  Relational Operator : RelationalOperator  Operator=<=  OutDataTypeStr=boolean  RndMeth=Nearest
  Switch : Switch  Criteria=u2 ~= 0
  y : Outport
  Dec? : Outport  Port=2
  wires:
  Relational Operator/1 -> Switch/2, Dec?/1
  u/1 -> Relational Operator/1, Switch/1
  Memory/1 -> Relational Operator/2, Switch/3
  Switch/1 -> Memory/1, y/1

== system NominalEncounter/Metrics/Common Metrics/Running Min Slant Range ==
  u : Inport
  MinMax : MinMax  Inputs=2
  Relational Operator : RelationalOperator  Operator=<=  OutDataTypeStr=boolean  RndMeth=Nearest
  Unit Delay : UnitDelay  InitialCondition=inf  SampleTime=-1
  min : Outport
  isMin : Outport  Port=2
  wires:
  Relational Operator/1 -> isMin/1
  Unit Delay/1 -> MinMax/2, Relational Operator/2  "old value"
  MinMax/1 -> Unit Delay/1, min/1
  u/1 -> Relational Operator/1, MinMax/1  "new value"

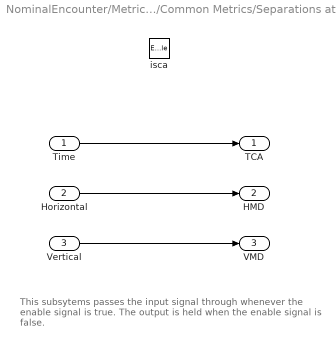
== system NominalEncounter/Metrics/Common Metrics/Separations at TCA ==
  note: This subsytems passes the input signal through whenever the enable signal is true. The output is held when the enable signal is false.
  Time : Inport
  Horizontal : Inport  Port=2
  Vertical : Inport  Port=3
  isca : EnablePort
  TCA : Outport
  HMD : Outport  Port=2
  VMD : Outport  Port=3
  wires:
  Time/1 -> TCA/1
  Horizontal/1 -> HMD/1
  Vertical/1 -> VMD/1

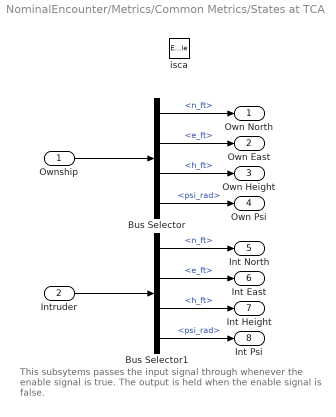
== system NominalEncounter/Metrics/Common Metrics/States at TCA ==
  note: This subsytems passes the input signal through whenever the enable signal is true. The output is held when the enable signal is false.
  Ownship : Inport
  Intruder : Inport  Port=2
  isca : EnablePort
  Bus Selector : BusSelector  OutputSignals=n_ft,e_ft,h_ft,psi_rad
  Bus Selector1 : BusSelector  OutputSignals=n_ft,e_ft,h_ft,psi_rad
  Own North : Outport
  Own East : Outport  Port=2
  Own Height : Outport  Port=3
  Own Psi : Outport  Port=4
  Int North : Outport  Port=5
  Int East : Outport  Port=6
  Int Height : Outport  Port=7
  Int Psi : Outport  Port=8
  wires:
  Ownship/1 -> Bus Selector/1
  Intruder/1 -> Bus Selector1/1
  Bus Selector/1 -> Own North/1  "<n_ft>"
  Bus Selector/2 -> Own East/1  "<e_ft>"
  Bus Selector/3 -> Own Height/1  "<h_ft>"
  Bus Selector1/1 -> Int North/1  "<n_ft>"
  Bus Selector1/2 -> Int East/1  "<e_ft>"
  Bus Selector1/3 -> Int Height/1  "<h_ft>"
  Bus Selector/4 -> Own Psi/1  "<psi_rad>"
  Bus Selector1/4 -> Int Psi/1  "<psi_rad>"

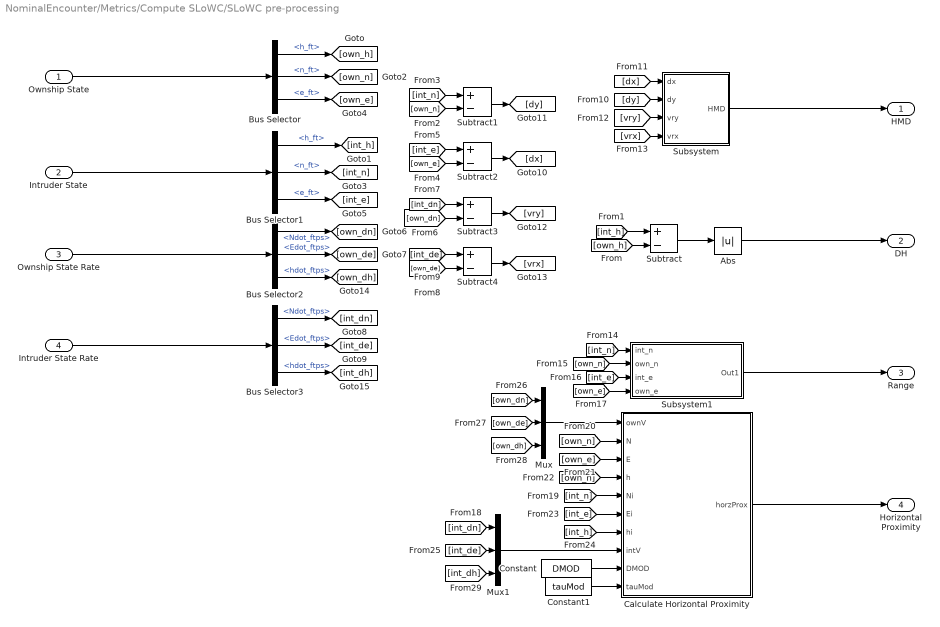
== system NominalEncounter/Metrics/Compute SLoWC/SLoWC pre-processing ==
  Ownship State : Inport
  Intruder State : Inport  Port=2
  Ownship State Rate : Inport  Port=3
  Intruder State Rate : Inport  Port=4
  Abs : Abs
  Bus Selector : BusSelector  OutputSignals=h_ft,n_ft,e_ft
  Bus Selector1 : BusSelector  OutputSignals=h_ft,n_ft,e_ft
  Bus Selector2 : BusSelector  OutputSignals=Ndot_ftps,Edot_ftps,hdot_ftps
  Bus Selector3 : BusSelector  OutputSignals=Ndot_ftps,Edot_ftps,hdot_ftps
  Calculate Horizontal Proximity : MATLAB Function  TreatAsAtomicUnit=on
  Constant : Constant  Value=DMOD
  Constant1 : Constant  Value=tauMod
  Mux : Mux  Inputs=3
  Mux1 : Mux  Inputs=3
  Subsystem : Subsystem
  Subsystem1 : Subsystem
  Subtract{,1..4} (5 alike) : Sum  Inputs=+-
  HMD : Outport
  DH : Outport  Port=2
  Range : Outport  Port=3
  Horizontal Proximity : Outport  Port=4
  wires:
  Subtract/1 -> Abs/1
  [own_dh] -> Mux/3
  Bus Selector/1 -> [own_h]  "<h_ft>"
  [own_dn] -> Subtract3/2
  Bus Selector1/3 -> [int_e]  "<e_ft>"
  [int_n] -> Calculate Horizontal Proximity/5(Ni)
  Bus Selector3/3 -> [int_dh]  "<hdot_ftps>"
  [int_h] -> Calculate Horizontal Proximity/7(hi)
  [int_e] -> Subtract2/1
  [own_h] -> Subtract/2
  Intruder State/1 -> Bus Selector1/1
  [own_n] -> Subtract1/2
  Constant/1 -> Calculate Horizontal Proximity/9(DMOD)
  [own_e] -> Subtract2/2
  [int_dh] -> Mux1/3
  Subtract4/1 -> [vrx]
  [int_h] -> Subtract/1
  Bus Selector1/1 -> [int_h]  "<h_ft>"
  [vry] -> Subsystem/3(vry)
  [own_n] -> Calculate Horizontal Proximity/2(N)
  Bus Selector3/1 -> [int_dn]  "<Ndot_ftps>"
  Subtract2/1 -> [dx]
  Bus Selector1/2 -> [int_n]  "<n_ft>"
  Bus Selector/2 -> [own_n]  "<n_ft>"
  Subtract3/1 -> [vry]
  [int_e] -> Subsystem1/3(int_e)
  [own_de] -> Mux/2
  Mux1/1 -> Calculate Horizontal Proximity/8(intV)
  Subtract1/1 -> [dy]
  [own_h] -> Calculate Horizontal Proximity/4(h)
  [dy] -> Subsystem/2(dy)
  [own_n] -> Subsystem1/2(own_n)
  [int_dn] -> Mux1/1
  Subsystem/1(HMD) -> HMD/1
  Bus Selector2/2 -> [own_de]  "<Edot_ftps>"
  [int_n] -> Subtract1/1
  Bus Selector2/3 -> [own_dh]  "<hdot_ftps>"
  [int_de] -> Subtract4/1
  Constant1/1 -> Calculate Horizontal Proximity/10(tauMod)
  Bus Selector/3 -> [own_e]  "<e_ft>"
  Subsystem1/1(Out1) -> Range/1
  [int_n] -> Subsystem1/1("int_n ")
  [int_e] -> Calculate Horizontal Proximity/6(Ei)
  [own_de] -> Subtract4/2
  Bus Selector3/2 -> [int_de]  "<Edot_ftps>"
  Mux/1 -> Calculate Horizontal Proximity/1(ownV)
  [dx] -> Subsystem/1("dx ")
  [int_dn] -> Subtract3/1
  Intruder State Rate/1 -> Bus Selector3/1
  [vrx] -> Subsystem/4(vrx)
  [own_dn] -> Mux/1
  Bus Selector2/1 -> [own_dn]  "<Ndot_ftps>"
  Abs/1 -> DH/1
  [own_e] -> Calculate Horizontal Proximity/3(E)
  Calculate Horizontal Proximity/1(horzProx) -> Horizontal Proximity/1
  Ownship State/1 -> Bus Selector/1
  [int_de] -> Mux1/2
  [own_e] -> Subsystem1/4(own_e)
  Ownship State Rate/1 -> Bus Selector2/1

== system NominalEncounter/Metrics/Common Metrics/Calculate Separations/Is NMAC ==
  minHorDist : Inport
  minVerDist : Inport  Port=2
  Abs2 : Abs
  Compare To Constant : simulink/Logic and Bit Operations/Compare To Constant  relop=<  const=500  OutDataTypeStr=boolean
  Compare To Constant1 : simulink/Logic and Bit Operations/Compare To Constant  relop=<  const=100  OutDataTypeStr=boolean
  Logical Operator : Logic  AllPortsSameDT=off  OutDataTypeStr=boolean
  NMAC : Outport
  wires:
  minHorDist/1 -> Compare To Constant/1
  minVerDist/1 -> Abs2/1
  Compare To Constant/1 -> Logical Operator/1
  Logical Operator/1 -> NMAC/1
  Compare To Constant1/1 -> Logical Operator/2
  Abs2/1 -> Compare To Constant1/1

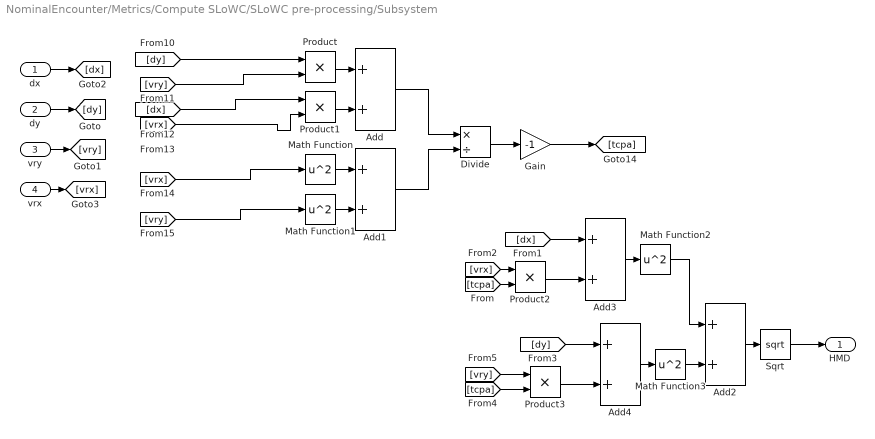
== system NominalEncounter/Metrics/Compute SLoWC/SLoWC pre-processing/Subsystem ==
  "dx " : Inport
  dy : Inport  Port=2
  vry : Inport  Port=3
  vrx : Inport  Port=4
  Add{,1..4} (5 alike) : Sum
  Divide : Product  Inputs=*/
  Gain : Gain  Gain=-1
  Math Function{,1..3} (4 alike) : Math  Operator=square  SaturateOnIntegerOverflow=on
  Product{,1..3} (4 alike) : Product
  Sqrt : Sqrt  SaturateOnIntegerOverflow=on
  HMD : Outport
  wires:
  Math Function1/1 -> Add1/2
  Gain/1 -> [tcpa]
  Add/1 -> Divide/1
  Math Function/1 -> Add1/1
  Product1/1 -> Add/2
  Product/1 -> Add/1
  [vrx] -> Math Function/1
  [vrx] -> Product1/2
  [dx] -> Product1/1
  Divide/1 -> Gain/1
  Add1/1 -> Divide/2
  [vry] -> Product/2
  [dy] -> Product/1
  [vry] -> Math Function1/1
  Sqrt/1 -> HMD/1
  Add2/1 -> Sqrt/1
  Math Function2/1 -> Add2/1
  Add3/1 -> Math Function2/1
  [dx] -> Add3/1
  [vrx] -> Product2/1
  Product2/1 -> Add3/2
  [tcpa] -> Product2/2
  Add4/1 -> Math Function3/1
  Math Function3/1 -> Add2/2
  Product3/1 -> Add4/2
  [dy] -> Add4/1
  [tcpa] -> Product3/2
  [vry] -> Product3/1
  "dx "/1 -> [dx]
  vrx/1 -> [vrx]
  vry/1 -> [vry]
  dy/1 -> [dy]

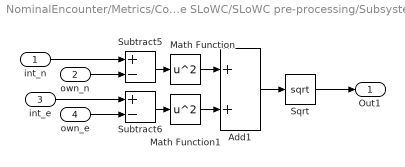
== system NominalEncounter/Metrics/Compute SLoWC/SLoWC pre-processing/Subsystem1 ==
  "int_n " : Inport
  own_n : Inport  Port=2
  int_e : Inport  Port=3
  own_e : Inport  Port=4
  Add1 : Sum
  Math Function : Math  Operator=square  SaturateOnIntegerOverflow=on
  Math Function1 : Math  Operator=square  SaturateOnIntegerOverflow=on
  Sqrt : Sqrt  SaturateOnIntegerOverflow=on
  Subtract5 : Sum  Inputs=+-
  Subtract6 : Sum  Inputs=+-
  Out1 : Outport
  wires:
  Math Function/1 -> Add1/1
  Add1/1 -> Sqrt/1
  Math Function1/1 -> Add1/2
  Subtract5/1 -> Math Function/1
  Sqrt/1 -> Out1/1
  Subtract6/1 -> Math Function1/1
  int_e/1 -> Subtract6/1
  own_n/1 -> Subtract5/2
  "int_n "/1 -> Subtract5/1
  own_e/1 -> Subtract6/2

== matlab function NominalEncounter/Metrics/Compute SLoWC/SLoWC pre-processing/Calculate Horizontal Proximity ==
  data: ownV input; N input; horzProx output; E input; h input; Ni input; Ei input; hi input; intV input; DMOD input; tauMod input
function horzProx = getHorzProx(ownV,N,E,h,Ni,Ei,hi,intV, DMOD, tauMod) 
% This block computes horizontal proximity (S_i in the Bihrle slide 3)

%Ri = [Ni-N; Ei-E; -(hi-h)];
Ri = [Ni-N; Ei-E; 0];

rangeRate = 0;

if(~isempty(Ri) && ~isempty(ownV) && ~isempty(intV))
    relVel = intV - ownV;
    rangeRate = dot(Ri/norm(Ri), relVel);
end

horzProx = max(DMOD, 0.5* (sqrt((rangeRate*tauMod)^2 + 4*DMOD^2) - rangeRate*tauMod) );
